simulink model "Clth_VD"  (R2016b)
settings: configuration reference "CodeGenConfigSet" (kept outside this file)
values from neighbouring files (symbols this model uses):
  Clth_nNoGearShftDet_C = Calibration.Parameter    [init_Clth_VD.m]
  Clth_tiGearShft_C = Calibration.Parameter    [init_Clth_VD.m]
  Clth_tiPlaDebDef_C = Calibration.Parameter    [init_Clth_VD.m]
  Clth_tiPlaDebOk_C = Calibration.Parameter    [init_Clth_VD.m]
  Clth_vNoGearShftDet_C = Calibration.Parameter    [init_Clth_VD.m]
  TRA_NUMGEAR_GEAR_NEUTR = int8(0)    [init_Clth_VD.m]
undefined symbols (not defined in the file or in its folder): Clth_VD_DT, SubSysExeState_conv
libraries: CXLib x5, simulink x1
settings Model: Creator=lenovo  LastModifiedBy=jiakui
settings ConfigSetRef: SourceLocation=Base Workspace

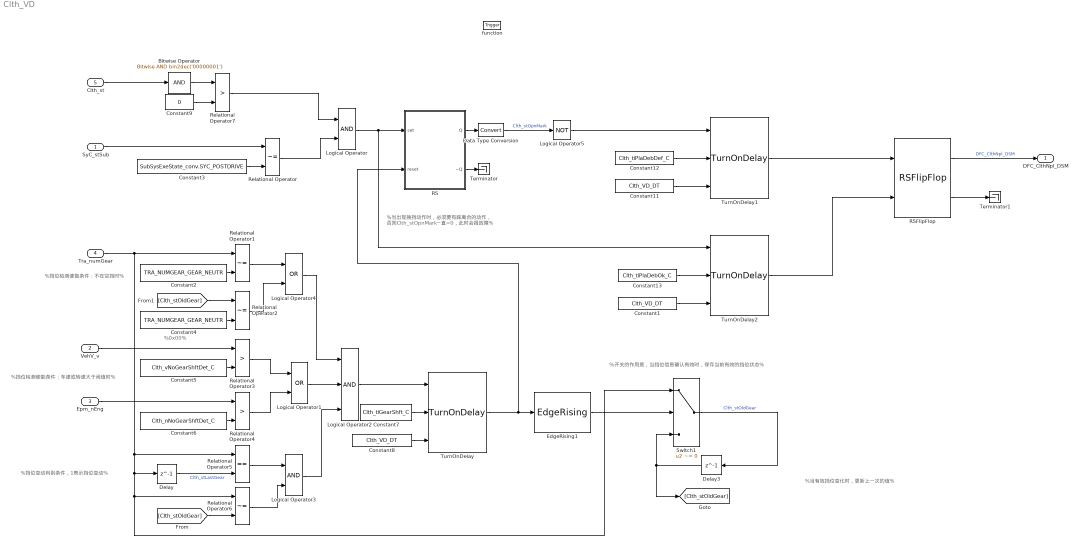
== system Clth_VD ==
  note: %0x00%
  note: %当出现换挡动作时，必须要有踩离合的动作，
      | 否则Clth_stOpnMark一直=0，此时会报故障%
  note: %开关的作用是，当挡位信息确认有效时，保存当前有效的挡位状态%
  note: %挡位检测使能条件：车速或转速大于阀值时%
  note: %挡位变动判别条件，1表示挡位变动%
  note: %挡位检测使能条件：不在空挡时%
  note: %当有效挡位变化时，更新上一次的值%
  SyC_stSub : Inport  Description=Current system/ECU sub-state  OutDataTypeStr=Enum: SubSysExeState_conv
  VehV_v : Inport  Tag=km/h  Description=Vehicle speed  Port=2  OutMin=0  OutMax=250  OutDataTypeStr=VehSpeed_km_h
  Epm_nEng : Inport  Tag=rpm  Description=Engine speed  Port=3  OutMin=0  OutMax=6000  OutDataTypeStr=EngSpeed_rpm
  Tra_numGear : Inport  Description=Current gear information  Port=4  OutMin=-128  OutMax=127  OutDataTypeStr=Tra_num
  Clth_st : Inport  Description=Clutch information  Port=5  OutMin=0  OutMax=255  OutDataTypeStr=State_uint8
  function : TriggerPort  TriggerType=function-call  VariantControl=Variant
  Bitwise Operator : simulink/Logic and Bit Operations/Bitwise Operator  logicop=AND  UseBitMask=on  BitMask=bin2dec('00000001')  BitMaskRealWorld=Stored Integer
  Constant1 : Constant  Value=Clth_VD_DT  OutDataTypeStr=Inherit: Inherit via back propagation  SampleTime=-1
  Constant11 : Constant  Value=Clth_VD_DT  OutDataTypeStr=Inherit: Inherit via back propagation  SampleTime=-1
  Constant12 : Constant  Value=Clth_tiPlaDebDef_C  SampleTime=-1
  Constant13 : Constant  Value=Clth_tiPlaDebOk_C  SampleTime=-1
  Constant2 : Constant  Value=TRA_NUMGEAR_GEAR_NEUTR  OutDataTypeStr=Inherit: Inherit via back propagation
  Constant3 : Constant  Value=SubSysExeState_conv.SYC_POSTDRIVE
  Constant4 : Constant  Value=TRA_NUMGEAR_GEAR_NEUTR  OutDataTypeStr=Inherit: Inherit via back propagation
  Constant5 : Constant  Value=Clth_vNoGearShftDet_C
  Constant6 : Constant  Value=Clth_nNoGearShftDet_C
  Constant7 : Constant  Value=Clth_tiGearShft_C
  Constant8 : Constant  Value=Clth_VD_DT  OutDataTypeStr=Inherit: Inherit via back propagation  SampleTime=-1
  Constant9 : Constant  Value=0  OutDataTypeStr=uint8
  Data Type Conversion : DataTypeConversion
  Delay : Delay  DelayLength=1  InitialCondition=0
  Delay3 : Delay  DelayLength=1  InitialCondition=0
  EdgeRising1 : CXLib/EdgeRising
  Logical Operator : Logic  RequirementInfo={'other' 'Clth_requirements.doc' '@Simulink_requirement_item_6' 'true' '离合器状态更改检测' '' } %GIDa_235f80fe_e9f0_4507_a0b2_7bb7f5a8dec5  AllPortsSameDT=off  OutDataTypeStr=boolean
  Logical Operator1 : Logic  RequirementInfo={'other' 'Clth_requirements.doc' '@Simulink_requirement_item_5' 'true' '档位状态更改需要满足相应的条件' '' } %GIDa_24f59ba5_46b3_4c18_9e6f_d8e0619c863b  Operator=OR  AllPortsSameDT=off  OutDataTypeStr=boolean
  Logical Operator2 : Logic  RequirementInfo={'other' 'Clth_requirements.doc' '@Simulink_requirement_item_5' 'true' '档位状态更改需要满足相应的条件' '' } %GIDa_67db322a_cfb8_4608_af64_a321660388c8  Inputs=3  AllPortsSameDT=off  OutDataTypeStr=boolean
  Logical Operator3 : Logic  RequirementInfo={'other' 'Clth_requirements.doc' '@Simulink_requirement_item_5' 'true' '档位状态更改需要满足相应的条件' '' } %GIDa_85785295_876f_4984_bdc7_e098ecd14462  AllPortsSameDT=off  OutDataTypeStr=boolean
  Logical Operator4 : Logic  RequirementInfo={'other' 'Clth_requirements.doc' '@Simulink_requirement_item_5' 'true' '档位状态更改需要满足相应的条件' '' } %GIDa_4295a9a3_a568_4fc5_afe0_3d1db1a54667  Operator=OR  AllPortsSameDT=off  OutDataTypeStr=boolean
  Logical Operator5 : Logic  Operator=NOT  AllPortsSameDT=off  OutDataTypeStr=boolean
  RS : Subsystem
  RSFlipFlop : CXLib/RSFlipFlop
  Relational Operator : RelationalOperator  Operator=~=  OutDataTypeStr=boolean  RndMeth=Simplest
  Relational Operator1 : RelationalOperator  RequirementInfo={'other' 'Clth_requirements.doc' '@Simulink_requirement_item_5' 'true' '档位状态更改需要满足相应的条件' '' } %GIDa_31d56d35_6466_4e5c_91cb_17ee97cf2648  Operator=~=  OutDataTypeStr=boolean  RndMeth=Simplest  InputSameDT=on
  Relational Operator2 : RelationalOperator  RequirementInfo={'other' 'Clth_requirements.doc' '@Simulink_requirement_item_5' 'true' '档位状态更改需要满足相应的条件' '' } %GIDa_d99faa96_6ecd_4bd9_aaf5_dd701b400a40  Operator=~=  OutDataTypeStr=boolean  RndMeth=Simplest  InputSameDT=on
  Relational Operator3 : RelationalOperator  RequirementInfo={'other' 'Clth_requirements.doc' '@Simulink_requirement_item_5' 'true' '档位状态更改需要满足相应的条件' '' } %GIDa_914094e7_5e4e_4659_8fa8_188232ccc662  Operator=>  OutDataTypeStr=boolean  RndMeth=Simplest  InputSameDT=on
  Relational Operator4 : RelationalOperator  RequirementInfo={'other' 'Clth_requirements.doc' '@Simulink_requirement_item_5' 'true' '档位状态更改需要满足相应的条件' '' } %GIDa_8d1c0ecb_9b2a_4dc5_8e46_5271d2899d16  Operator=>  OutDataTypeStr=boolean  RndMeth=Simplest  InputSameDT=on
  Relational Operator5 : RelationalOperator  RequirementInfo={'other' 'Clth_requirements.doc' '@Simulink_requirement_item_5' 'true' '档位状态更改需要满足相应的条件' '' } %GIDa_84687ae1_8cc2_4bb0_a97b_2ef2da8efda5  Operator===  OutDataTypeStr=boolean  RndMeth=Simplest  InputSameDT=on
  Relational Operator6 : RelationalOperator  RequirementInfo={'other' 'Clth_requirements.doc' '@Simulink_requirement_item_5' 'true' '档位状态更改需要满足相应的条件' '' } %GIDa_ea93e732_ea69_45ac_8307_189ee3141526  Operator=~=  OutDataTypeStr=boolean  RndMeth=Simplest
  Relational Operator7 : RelationalOperator  Operator=>  OutDataTypeStr=boolean  RndMeth=Simplest  InputSameDT=on
  Switch1 : Switch  Criteria=u2 ~= 0  OutDataTypeStr=Inherit: Inherit via back propagation  InputSameDT=on
  Terminator : Terminator
  Terminator1 : Terminator
  TurnOnDelay : CXLib/TurnOnDelay
  TurnOnDelay1 : CXLib/TurnOnDelay  RequirementInfo={'other' 'Clth_requirements.doc' '@Simulink_requirement_item_7' 'true' '离合器故障处理' '' } %GIDa_dc07ae57_516b_4b4d_93dc_848d7aac72b8
  TurnOnDelay2 : CXLib/TurnOnDelay  RequirementInfo={'other' 'Clth_requirements.doc' '@Simulink_requirement_item_7' 'true' '离合器故障处理' '' } %GIDa_3d40c361_86ca_49a5_a2ac_dd868482ceaf
  DFC_ClthNpl_DSM : Outport  Description="state of error \"DFC_ClthNpl\""  OutMin=0  OutMax=1  OutDataTypeStr=boolean
  wires:
  RSFlipFlop/1 -> DFC_ClthNpl_DSM/1  "DFC_ClthNpl_DSM"
  Constant8/1 -> TurnOnDelay/3
  Data Type Conversion/1 -> Logical Operator5/1  "Clth_stOpnMark"
  RS/2(~Q) -> Terminator/1
  Delay3/1 -> Switch1/3, [Clth_stOldGear]
  Switch1/1 -> Delay3/1  "Clth_stOldGear"
  Tra_numGear/1 -> Relational Operator1/1, Relational Operator5/1, Delay/1, Relational Operator6/1, Switch1/1
  RS/1(Q) -> Data Type Conversion/1
  Bitwise Operator/1 -> Relational Operator7/1
  Constant9/1 -> Relational Operator7/2
  TurnOnDelay/1 -> RS/2(reset), EdgeRising1/1
  [Clth_stOldGear] -> Relational Operator2/1
  [Clth_stOldGear] -> Relational Operator6/2
  EdgeRising1/1 -> Switch1/2
  Constant7/1 -> TurnOnDelay/2
  Logical Operator2/1 -> TurnOnDelay/1
  Logical Operator3/1 -> Logical Operator2/3
  Logical Operator4/1 -> Logical Operator2/1
  Relational Operator2/1 -> Logical Operator4/2
  Relational Operator1/1 -> Logical Operator4/1
  Relational Operator5/1 -> Logical Operator3/1
  Relational Operator6/1 -> Logical Operator3/2
  Logical Operator1/1 -> Logical Operator2/2
  Delay/1 -> Relational Operator5/2  "Clth_stLastGear"
  Relational Operator4/1 -> Logical Operator1/2
  Relational Operator3/1 -> Logical Operator1/1
  Epm_nEng/1 -> Relational Operator4/1
  Constant6/1 -> Relational Operator4/2
  VehV_v/1 -> Relational Operator3/1
  Constant5/1 -> Relational Operator3/2
  Constant4/1 -> Relational Operator2/2
  Constant2/1 -> Relational Operator1/2
  Relational Operator/1 -> Logical Operator/2
  Relational Operator7/1 -> Logical Operator/1
  Constant3/1 -> Relational Operator/2
  SyC_stSub/1 -> Relational Operator/1
  Clth_st/1 -> Bitwise Operator/1
  Constant11/1 -> TurnOnDelay1/3
  Constant1/1 -> TurnOnDelay2/3
  Logical Operator/1 -> TurnOnDelay2/1, RS/1(set)
  Constant12/1 -> TurnOnDelay1/2
  Constant13/1 -> TurnOnDelay2/2
  TurnOnDelay1/1 -> RSFlipFlop/1
  TurnOnDelay2/1 -> RSFlipFlop/2
  Logical Operator5/1 -> TurnOnDelay1/1
  RSFlipFlop/2 -> Terminator1/1

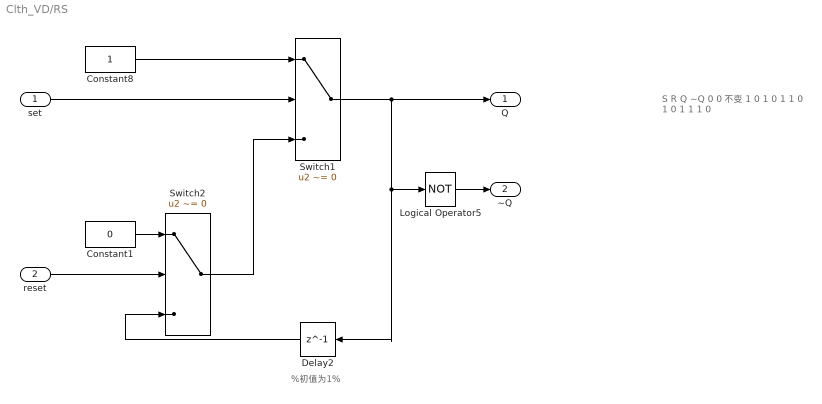
== system Clth_VD/RS ==
  note: S
      | R
      | Q
      | ~Q
      |
      | 0
      | 0
      | 不变
      | 1
      |
      | 0
      | 1
      | 0
      | 1
      |
      | 1
      | 0
      | 1
      | 0
      |
      | 1
      | 1
      | 1
      | 0
  note: %初值为1%
  set : Inport
  reset : Inport  Port=2
  Constant1 : Constant  Value=0  OutDataTypeStr=boolean
  Constant8 : Constant  OutDataTypeStr=boolean
  Delay2 : Delay  DelayLength=1  InitialCondition=1
  Logical Operator5 : Logic  Operator=NOT  AllPortsSameDT=off  OutDataTypeStr=boolean
  Switch1 : Switch  Criteria=u2 ~= 0  OutDataTypeStr=Inherit: Inherit via back propagation  InputSameDT=on
  Switch2 : Switch  Criteria=u2 ~= 0  OutDataTypeStr=Inherit: Inherit via back propagation  InputSameDT=on
  Q : Outport
  ~Q : Outport  Port=2
  wires:
  Delay2/1 -> Switch2/3
  Switch2/1 -> Switch1/3
  Constant1/1 -> Switch2/1
  Constant8/1 -> Switch1/1
  Switch1/1 -> Q/1, Delay2/1, Logical Operator5/1
  Logical Operator5/1 -> ~Q/1
  set/1 -> Switch1/2
  reset/1 -> Switch2/2
